simulink model "SafetyCriticalLQR"  (R2020b)
settings: Solver=VariableStepAuto  StartTime=0.0  StopTime=tf_upperbound  RelTol=1e-7
PreLoadFcn:
  | SafetyCriticalLQRParams
values from neighbouring files (symbols this model uses):
  A = [0  1; 0  0]    [CBFExample.mat]    (also in CBFExample_DifferentEta.mat; SafetyCriticalLQRParams.m = [0 1;0 0])
  B = [0 1]    [CBFExample.mat]    (also in CBFExample_DifferentEta.mat; SafetyCriticalLQRParams.m = [0; 1])
  C = [1  0; 0  1]    [CBFExample.mat]    (also in CBFExample_DifferentEta.mat; SafetyCriticalLQRParams.m = eye(Nx))
  cT = [10 -5]    [CBFExample.mat]    (also in CBFExample_DifferentEta.mat; SafetyCriticalLQRParams.m = [10;-5])
  D = [0 0]    [CBFExample.mat]    (also in CBFExample_DifferentEta.mat; SafetyCriticalLQRParams.m = [0;0])
  eta = 2    [CBFExample.mat]    (also in CBFExample_DifferentEta.m = etaAll(i); CBFExample_DifferentEta.mat; SafetyCriticalLQRParams.m)
  filterCase = 2    [CBFExample.m]    (also in CBFExample.mat; CBFExample_DifferentEta.m; CBFExample_DifferentEta.mat; SafetyCriticalLQRParams.m = 1)
  K = [0.316227766017 0.855836159574]    [CBFExample.mat]    (also in CBFExample_DifferentEta.mat)
  P = [1.35319578409  1.58113883008; 1.58113883008  4.27918079787]    [CBFExample.mat]    (also in CBFExample_DifferentEta.mat)
  Ref = [0 0]    [CBFExample.mat]    (also in CBFExample_DifferentEta.mat; SafetyCriticalLQRParams.m = [0;0])
  rT = 4    [CBFExample.mat]    (also in CBFExample_DifferentEta.mat; SafetyCriticalLQRParams.m)
  x0 = [10 10]    [CBFExample.mat]    (also in CBFExample_DifferentEta.mat; SafetyCriticalLQRParams.m = [10;10])
libraries: simulink x2
settings Model: Creator=Jyot Buch  LastModifiedBy=Jyot Buch

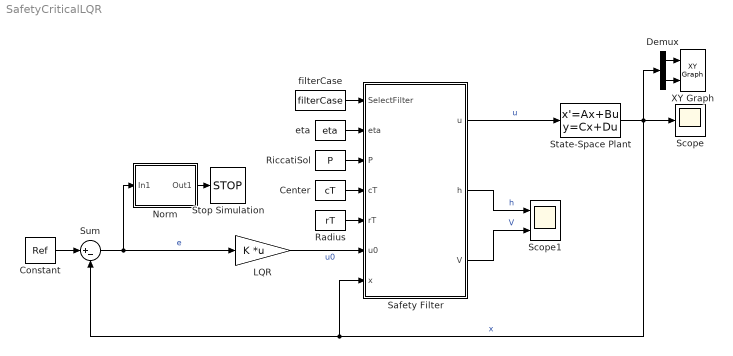
== system SafetyCriticalLQR ==
  Center : Constant  Value=cT
  Constant : Constant  Value=Ref
  Demux : Demux  Outputs=2
  LQR : Gain  Gain=K  Multiplication=Matrix(K*u) (u vector)
  Norm : Subsystem
  Radius : Constant  Value=rT
  RiccatiSol : Constant  Value=P
  Safety Filter : MATLAB Function  TreatAsAtomicUnit=on
  Scope : Scope
  Scope1 : Scope  NumInputPorts=2
  State-Space Plant : StateSpace  A=A  B=B  C=C  D=D  InitialCondition=x0
  Stop Simulation : Stop
  Sum : Sum  Inputs=|+-
  XY Graph : simulink/Sinks/XY Graph  xmin=-20  xmax=20  ymin=-15  ymax=15  st=-1
  eta : Constant  Value=eta
  filterCase : Constant  Value=filterCase
  wires:
  State-Space Plant/1 -> Safety Filter/7(x), Sum/2, Scope/1, Demux/1  "x"
  Constant/1 -> Sum/1
  Sum/1 -> LQR/1, Norm/1(In1)  "e"
  LQR/1 -> Safety Filter/6(u0)  "u0"
  Safety Filter/1(u) -> State-Space Plant/1  "u"
  Radius/1 -> Safety Filter/5(rT)
  Demux/2 -> XY Graph/2
  Demux/1 -> XY Graph/1
  filterCase/1 -> Safety Filter/1(SelectFilter)
  Center/1 -> Safety Filter/4(cT)
  RiccatiSol/1 -> Safety Filter/3(P)
  Safety Filter/2(h) -> Scope1/1  "h"
  Safety Filter/3(V) -> Scope1/2  "V"
  Norm/1(Out1) -> Stop Simulation/1
  eta/1 -> Safety Filter/2(eta)

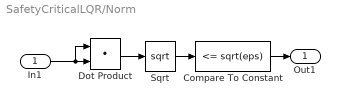
== system SafetyCriticalLQR/Norm ==
  In1 : Inport
  Compare To Constant : simulink/Logic and Bit Operations/Compare To Constant  relop=<=  const=sqrt(eps)  OutDataTypeStr=boolean
  Dot Product : DotProduct  InputSameDT=on  OutDataTypeStr=Inherit: Inherit via internal rule
  Sqrt : Sqrt  SaturateOnIntegerOverflow=on
  Out1 : Outport
  wires:
  In1/1 -> Dot Product/1, Dot Product/2
  Dot Product/1 -> Sqrt/1
  Sqrt/1 -> Compare To Constant/1
  Compare To Constant/1 -> Out1/1

== matlab function SafetyCriticalLQR/Safety Filter ==
  data: SelectFilter input; eta input; P input; cT input; rT input; u0 input; u output; x input; h output; V output
function [u,h,V] = fcn(SelectFilter,eta,P,cT,rT,u0,x)

% Compute h and V
h = (x(1)-cT(1))^2 + (x(2)-cT(2))^2 - rT^2;
V = x'*P*x;

% Select filter based on the specified case
switch SelectFilter
    case 1
        % Nominal LQR
        u = u0;
        
    case 2
        % CBF Only
        u = LOCALCBFQP(eta,h,cT,u0,x);
        
    otherwise
        % Openloop
        u = u0*0;
end
end

%% LOCALCBFQP
function u = LOCALCBFQP(eta,h,cT,u0,x)
% Inequality Safety Constraints for QP
% Aineq'*u <= bineq
Aineq = -2*(x(2)-cT(2));
bineq = 2*(x(1)-cT(1))*x(2) + eta*h;

% Solve QP
SolveQPCase = 1;
switch SolveQPCase
    case 1
        % Numerical Solution
        H = 1;
        f = -u0;
        opt = optimoptions('quadprog','Algorithm','active-set','Display','off');
        u = quadprog(H,f,Aineq,bineq,[],[],[],[],u0,opt);
        
    case 2
        % Explicit Solution
        rho = -bineq+Aineq*u0;
        if rho<=0
            zopt = 0;
        else
            zopt = -rho*Aineq/Aineq^2;
        end
        u = zopt+u0;
end
end
